simulink model "Step_04"  (Simulink 7.9)
settings: Solver=ode23  StartTime=0.0  StopTime=100  MaxStep=1  RelTol=1e-3
libraries: simulink x1
settings Model: Creator=wcampbel  LastModifiedBy=wcampbel
settings DebuggingCC: FcnCallInpInsideContextMsg=Use local settings  StrictBusMsg=Warning
settings GRTTargetCC: CombineOutputUpdateFcns=off  GRTInterface=on

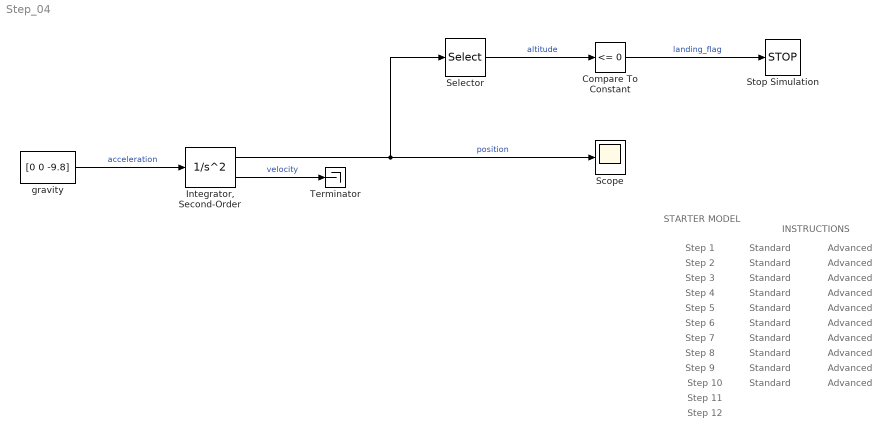
== system Step_04 ==
  note: Step 1
  note: Step 2
  note: Step 3
  note: STARTER
      | MODEL
  note: INSTRUCTIONS
  note: Step 4
  note: Step 5
  note: Step 6
  note: Standard
  note: Advanced
  note: Standard
  note: Advanced
  note: Standard
  note: Advanced
  note: Standard
  note: Standard
  note: Advanced
  note: Standard
  note: Advanced
  note: Step 7
  note: Step 8
  note: Step 9
  note: Step 10
  note: Step 11
  note: Standard
  note: Advanced
  note: Advanced
  note: Advanced
  note: Advanced
  note: Standard
  note: Standard
  note: Standard
  note: Advanced
  note: Step 12
  Compare To Constant : simulink/Logic and Bit Operations/Compare To Constant  relop=<=  const=0  OutDataTypeStr=boolean
  "Integrator, Second-Order" : SecondOrderIntegrator  ICX=[0 0 500]  ICDXDT=[8 -10 5]
  Scope : Scope
      settings: ShowLegends=on  TimeRange=12  YMin=-200  YMax=600
  Selector : Selector  InputPortWidth=3  IndexOptions=Index vector (dialog)  Indices=3  OutputSizes=1
  Stop Simulation : Stop
  Terminator : Terminator
  gravity : Constant  Value=[0 0 -9.8]
  wires:
  gravity/1 -> "Integrator, Second-Order"/1  "acceleration"
  Selector/1 -> Compare To Constant/1  "altitude"
  "Integrator, Second-Order"/1 -> Scope/1, Selector/1  "position"
  "Integrator, Second-Order"/2 -> Terminator/1  "velocity"
  Compare To Constant/1 -> Stop Simulation/1  "landing_flag"
